simulink model "mconversion12"  (Simulink 6.0)
settings: Solver=ode3  StartTime=0.0  StopTime=10.0  RelTol=1e-3
libraries: mylib x2
settings Model: Creator=awarlock  LastModifiedBy=awarlock  ExtModeAutoUpdateStatusClock=off
settings OptimizationCC: InlineParams=on
settings DebuggingCC: CheckExecutionContextPreStartOutputMsg=on  CheckExecutionContextRuntimeOutputMsg=on  SolverPrmCheckMsg=none
settings SFSimCC: SFSimApplyToAllLibs=on  SFSimBuildMode=Incremental

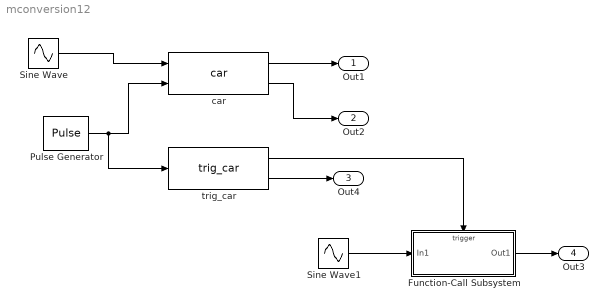
== system mconversion12 ==
  Function-Call Subsystem : Subsystem  TreatAsAtomicUnit=on  PropExecContextAcrossSSBoundary=on
  Pulse Generator : DiscretePulseGenerator  PulseType=Time based  PulseWidth=50
  Sine Wave : Sin  SampleTime=0
  Sine Wave1 : Sin  SampleTime=0
  car : mylib/car
  trig_car : mylib/trig_car
  Out1 : Outport
  Out2 : Outport  Port=2
  Out4 : Outport  Port=3
  Out3 : Outport  Port=4
  wires:
  Sine Wave/1 -> car/1
  Pulse Generator/1 -> car/2, trig_car/1
  car/1 -> Out1/1
  car/2 -> Out2/1
  trig_car/1 -> Function-Call Subsystem/Trigger
  trig_car/2 -> Out4/1
  Function-Call Subsystem/1(Out1) -> Out3/1
  Sine Wave1/1 -> Function-Call Subsystem/1(In1)

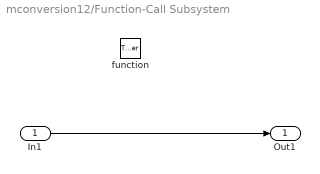
== system mconversion12/Function-Call Subsystem ==
  In1 : Inport  LatchInput=off
  function : TriggerPort  TriggerType=function-call
  Out1 : Outport
  wires:
  In1/1 -> Out1/1
